simulink model "MPCtest"  (R2021b)
settings: Solver=VariableStepAuto  StartTime=0.0  StopTime=60  RelTol=1e-3
libraries: dspnetwork x2, sldrtlib x1
settings Model: Creator=Kuorun Liu  LastModifiedBy=Kuorun Liu

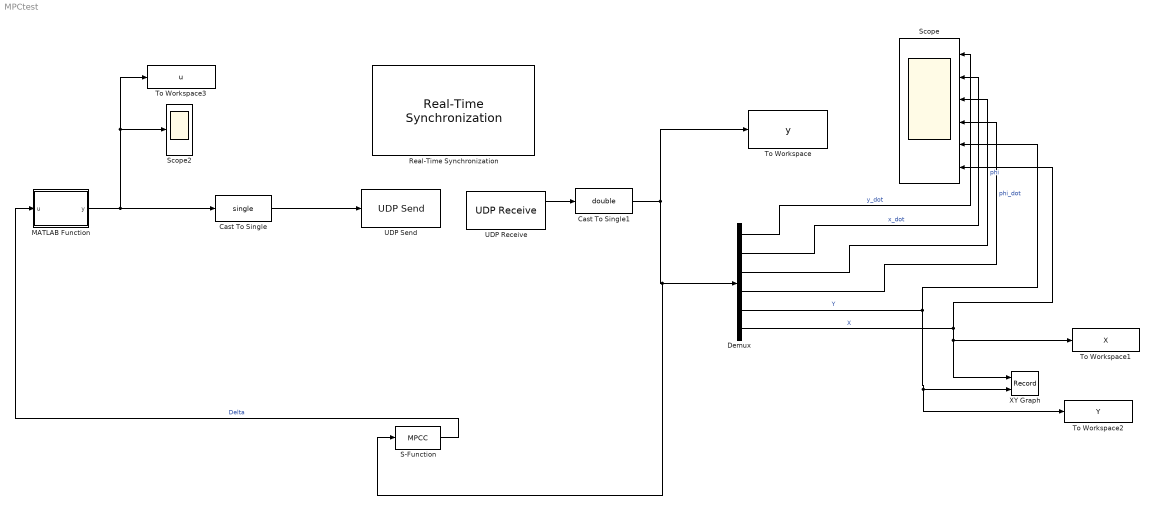
== system MPCtest ==
  Cast To Single : DataTypeConversion  OutDataTypeStr=single
  Cast To Single1 : DataTypeConversion  OutDataTypeStr=double
  Demux : Demux  Outputs=6
  MATLAB Function : MATLAB Function  TreatAsAtomicUnit=on
  Real-Time Synchronization : sldrtlib/Real-Time Synchronization  SampleTime=0.0005  MaxMissedTicks=10000  ShowMissedTicks=off  YieldWhenWaiting=off
  S-Function : S-Function  FunctionName=MPCC  SFunctionDeploymentMode=off  EnableBusSupport=off
  Scope : Scope  NumInputPorts=6
  Scope2 : Scope
  To Workspace : ToWorkspace  VariableName=y  SampleTime=-1
  To Workspace1 : ToWorkspace  VariableName=X  SampleTime=-1
  To Workspace2 : ToWorkspace  VariableName=Y  SampleTime=-1
  To Workspace3 : ToWorkspace  VariableName=u  SampleTime=-1
  UDP Receive : dspnetwork/UDP Receive  localURL='0.0.0.0'  localPort=2241  remoteURL='0.0.0.0'  remotePort=-1  recvBufferSize=8192  dims=6  signalDatatype=single  isComplex=off  isVarSize=off  showBlockingTime=off  blockingTime=0  sampletime=0.0005  blockPlatform=[]
  UDP Send : dspnetwork/UDP Send  remoteURL='127.0.0.1'  remotePort=2240  localURL='0.0.0.0'  localPortSource=Automatically determine  localPort=-1  sendBufferSize=8192  sampletime=-1  blockPlatform=[]  separateLengthPort=0
  XY Graph : Record  FileSettingsInternal="{\"entries\":[{\"content\":{\"excelSettings\":{\"content\":{},\"type\":\"Streamout.ExcelSettings\"}},\"type\":\"Streamout.FileSettingStorage\",\"uuid\":\"d49a2cb3-4dd4-4d4c-a4d3-4cefe22dc661\"}],\"packageUris\":[\"http://schema.mathworks.com/mf0/streamout_blocks/R2020a\"],\"version\":\"1.0\"}"  Layout=[1 1]  SignalsInternal="{\"entries\":[{\"content\":{\"signals\":[{\"content\":{\"blockPath\":[\"MPCtest/XY Graph\"],\"channel\":[],\"dimensions\":[1,1],\"domain\":\"MPCtest/XY Graph\",\"lineColor\":\"#0072bd\",\"plots\":[1],\"port\":1,\"sid\":[\"\"],\"signalID\":5878,\"signalName\":\"X\"},\"type\":\"RecordBlkView.Signal\",\"uuid\":\"0fe85bda-62a6-4950-a2ad-169c7f0b23ac\"},{\"content\":{\"blockPath\":[\"MPCtest/XY Graph\"],\"channel\":[],\"dimensions\":[1,1],\"domain\":\"MPCtest/XY Graph\",\"lineColor\":\"#0072bd\",\"plots\":[1],\"port\":2,\"sid\":[\"\"],\"signalID\":5882,\"signalName\":\"Y\"},\"type\":\"RecordBlkView.Signal\",\"uuid\":\"81c73132-6309-4e38-bc64-f7388e73532b\"}]},\"type\":\"RecordBlkView.InputSignals\",\"uuid\":\"772e764a-068b-41f8-8c60-aab052911c54\"}],\"packageUris\":[\"http://schema.mathworks.com/mf0/streamout_blocks/R2020a\"],\"version\":\"1.0\"}"  VisualizationBindings="{\"xyplotplugin\":{\"info\":[{\"series\":[{\"bindingParametersList\":[{\"parameter\":\"X-Axis\",\"signalID\":5878,\"signalName\":\"X\"},{\"parameter\":\"Y-Axis\",\"signalID\":5882,\"signalName\":\"Y\"}],\"seriesID\":647}],\"subplotID\":1}]}}"  CompatibilityTag=XY
  wires:
  UDP Receive/1 -> Cast To Single1/1
  Demux/1 -> Scope/1  "y_dot"
  Demux/2 -> Scope/2  "x_dot"
  Demux/3 -> Scope/3  "phi"
  Demux/4 -> Scope/4  "phi_dot"
  Demux/5 -> Scope/5, To Workspace2/1, XY Graph/2  "Y"
  Demux/6 -> Scope/6, To Workspace1/1, XY Graph/1  "X"
  S-Function/1 -> MATLAB Function/1(u)  "Delta"
  MATLAB Function/1(y) -> To Workspace3/1, Scope2/1, Cast To Single/1
  Cast To Single/1 -> UDP Send/1
  Cast To Single1/1 -> S-Function/1, Demux/1, To Workspace/1

== matlab function MPCtest/MATLAB Function ==
  data: u input; y output
function y = fcn(u)
%y=1.6372*u;
y=2*u;
